simulink model "BlockDiagram_Detailed_Fluids_FirstPrinc"  (R2025b)
settings: Solver=VariableStepAuto  StartTime=0.0  StopTime=10.0  RelTol=1e-3
values from neighbouring files (symbols this model uses):
  c_star_vec = [ ... (first row only)    [cstar_lookup_table.m]
  P_c_vec = 270:350    [a_lookup_table.m]    (also in cstar_lookup_table.m)
undefined symbols (not defined in the file or in its folder): CdA_inj_ox, CdA_max_valve_ox, P_amb, P_feed_f, P_feed_ox, rho_f, rho_ox, V_c
settings Model: Creator=gruby  LastModifiedBy=gruby

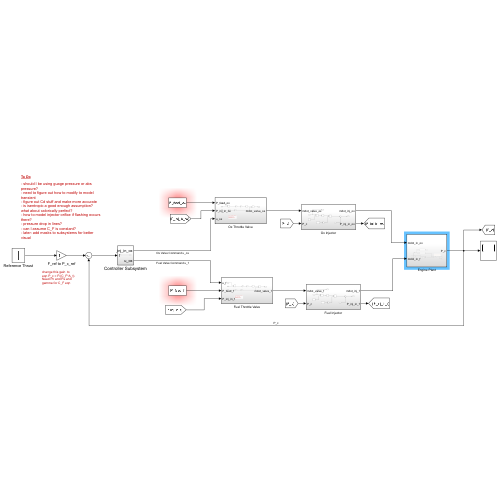
[thumbnail: Simulink's stored preview of the top-level diagram]
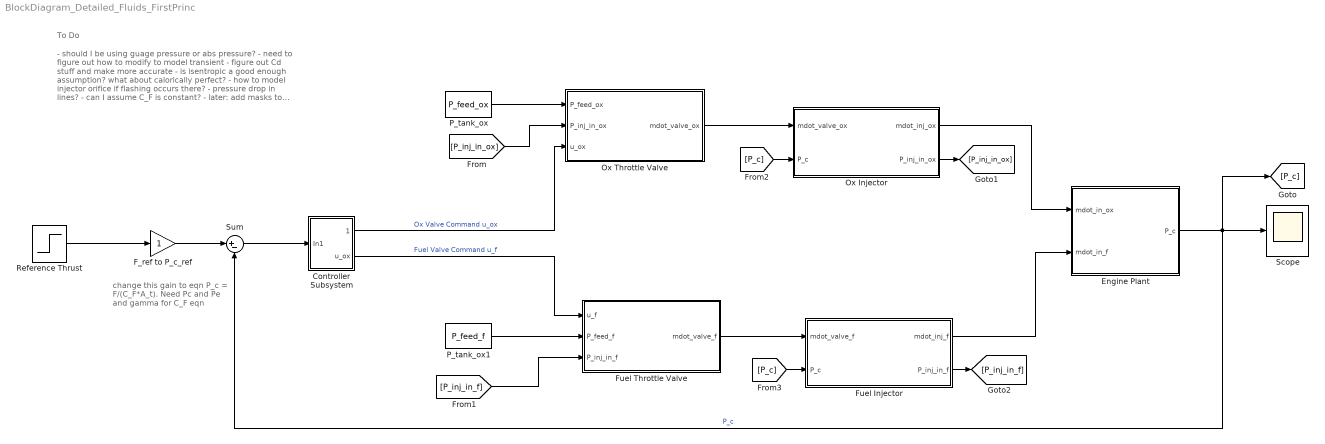
== system BlockDiagram_Detailed_Fluids_FirstPrinc ==
  note: To Do
  note: - should I be using guage pressure or abs pressure?
      | - need to figure out how to modify to model transient
      | - figure out Cd stuff and make more accurate
      | - is isentropic a good enough assumption? what about calorically perfect?
      | - how to model injector orifice if flashing occurs there?
      | - pressure drop in lines?
      | - can I assume C_F is constant?
      | - later: add masks to subsystems for better visual
  note: change this gain to eqn P_c = F/(C_F*A_t). Need Pc and Pe and gamma for C_F eqn
  Controller Subsystem : Subsystem
  Engine Plant : Subsystem
  F_ref to P_c_ref : Gain
  Fuel Injector : Subsystem
  Fuel Throttle Valve : Subsystem
  Ox Injector : Subsystem
  Ox Throttle Valve : Subsystem
  P_tank_ox : Constant  Value=P_feed_ox
  P_tank_ox1 : Constant  Value=P_feed_f
  Reference Thrust : Step  SampleTime=0
  Scope : Scope
      settings: ActiveDisplayYMinimum=-1.8374784378622904  ActiveDisplayYMaximum=16.537497604206919
  Sum : Sum  Inputs=|+-
  wires:
  Sum/1 -> Controller Subsystem/1(In1)
  F_ref to P_c_ref/1 -> Sum/1
  Reference Thrust/1 -> F_ref to P_c_ref/1
  Engine Plant/1(P_c) -> Scope/1, [P_c], Sum/2  "P_c"
  [P_c] -> Ox Injector/2(P_c)
  Controller Subsystem/1(P_inj_in_ox) -> Ox Throttle Valve/3(u_ox)  "Ox Valve Command u_ox"
  P_tank_ox/1 -> Ox Throttle Valve/1(P_feed_ox)
  Ox Throttle Valve/1(mdot_valve_ox) -> Ox Injector/1(mdot_valve_ox)
  Ox Injector/1(mdot_inj_ox) -> Engine Plant/1(mdot_in_ox)
  [P_inj_in_ox] -> Ox Throttle Valve/2(P_inj_in_ox)
  Ox Injector/2(P_inj_in_ox) -> [P_inj_in_ox]
  Controller Subsystem/2(u_ox) -> Fuel Throttle Valve/1(u_f)  "Fuel Valve Command u_f"
  Fuel Injector/2(P_inj_in_f) -> [P_inj_in_f]
  [P_inj_in_f] -> Fuel Throttle Valve/3(P_inj_in_f)
  Fuel Injector/1(mdot_inj_f) -> Engine Plant/2(mdot_in_f)
  [P_c] -> Fuel Injector/2(P_c)
  Fuel Throttle Valve/1(mdot_valve_f) -> Fuel Injector/1(mdot_valve_f)
  P_tank_ox1/1 -> Fuel Throttle Valve/2(P_feed_f)

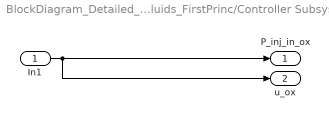
== system BlockDiagram_Detailed_Fluids_FirstPrinc/Controller Subsystem ==
  In1 : Inport
  P_inj_in_ox : Outport
  u_ox : Outport  Port=2
  wires:
  In1/1 -> u_ox/1, P_inj_in_ox/1

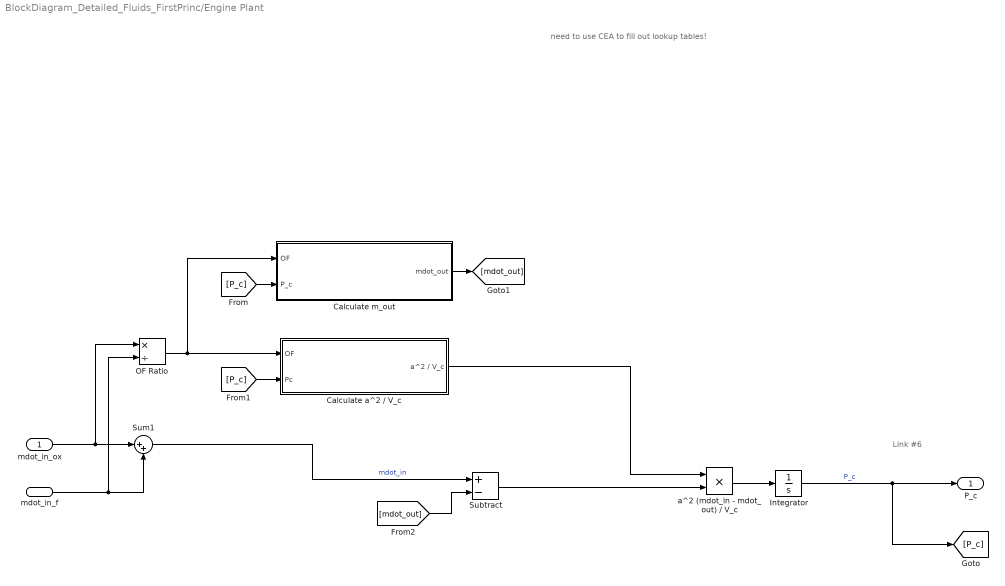
== system BlockDiagram_Detailed_Fluids_FirstPrinc/Engine Plant ==
  note: Link #6
  note: need to use CEA to fill out lookup tables!
  mdot_in_ox : Inport
  mdot_in_f : Inport  Port=2
  Calculate a^2 / V_c : Subsystem
  Calculate m_out : Subsystem
  Integrator : Integrator  InitialCondition=P_amb
  OF Ratio : Product  Inputs=*/
  Subtract : Sum  Inputs=+-
  Sum1 : Sum  Inputs=|++
  "a^2 (mdot_in - mdot_out) / V_c " : Product
  P_c : Outport
  wires:
  mdot_in_f/1 -> OF Ratio/2, Sum1/2
  mdot_in_ox/1 -> OF Ratio/1, Sum1/1
  Integrator/1 -> [P_c], P_c/1  "P_c"
  OF Ratio/1 -> Calculate m_out/1(OF), Calculate a^2 / V_c/1(OF)
  "a^2 (mdot_in - mdot_out) / V_c "/1 -> Integrator/1
  [P_c] -> Calculate m_out/2(P_c)
  [P_c] -> Calculate a^2 / V_c/2(Pc)
  Calculate a^2 / V_c/1(a^2 / V_c) -> "a^2 (mdot_in - mdot_out) / V_c "/1
  Calculate m_out/1(mdot_out) -> [mdot_out]
  Sum1/1 -> Subtract/1  "mdot_in"
  [mdot_out] -> Subtract/2
  Subtract/1 -> "a^2 (mdot_in - mdot_out) / V_c "/2

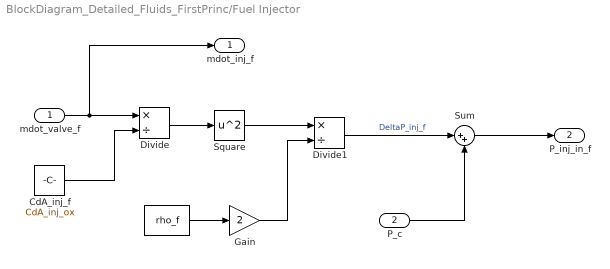
== system BlockDiagram_Detailed_Fluids_FirstPrinc/Fuel Injector ==
  mdot_valve_f : Inport
  P_c : Inport  Port=2
  "   " : Constant  Value=rho_f
  CdA_inj_f : Constant  Value=CdA_inj_ox
  Divide : Product  Inputs=*/
  Divide1 : Product  Inputs=*/
  Gain : Gain  Gain=2
  Square : Math  Operator=square
  Sum : Sum  Inputs=|++
  mdot_inj_f : Outport
  P_inj_in_f : Outport  Port=2
  wires:
  mdot_valve_f/1 -> mdot_inj_f/1, Divide/1
  CdA_inj_f/1 -> Divide/2
  Divide/1 -> Square/1
  Gain/1 -> Divide1/2
  "   "/1 -> Gain/1
  Square/1 -> Divide1/1
  Divide1/1 -> Sum/1  "DeltaP_inj_f"
  P_c/1 -> Sum/2
  Sum/1 -> P_inj_in_f/1

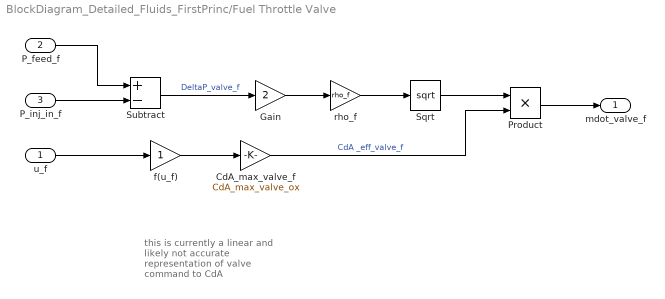
== system BlockDiagram_Detailed_Fluids_FirstPrinc/Fuel Throttle Valve ==
  note: this is currently a linear and likely not accurate representation of valve command to CdA
  u_f : Inport
  P_feed_f : Inport  Port=2
  P_inj_in_f : Inport  Port=3
  CdA_max_valve_f : Gain  Gain=CdA_max_valve_ox
  Gain : Gain  Gain=2
  Product : Product
  Sqrt : Sqrt
  Subtract : Sum  Inputs=+-
  f(u_f) : Gain
  rho_f : Gain  Gain=rho_f
  mdot_valve_f : Outport
  wires:
  f(u_f)/1 -> CdA_max_valve_f/1
  u_f/1 -> f(u_f)/1
  CdA_max_valve_f/1 -> Product/2  "CdA _eff_valve_f"
  P_feed_f/1 -> Subtract/1
  Subtract/1 -> Gain/1  "DeltaP_valve_f"
  Gain/1 -> rho_f/1
  rho_f/1 -> Sqrt/1
  Sqrt/1 -> Product/1
  Product/1 -> mdot_valve_f/1
  P_inj_in_f/1 -> Subtract/2

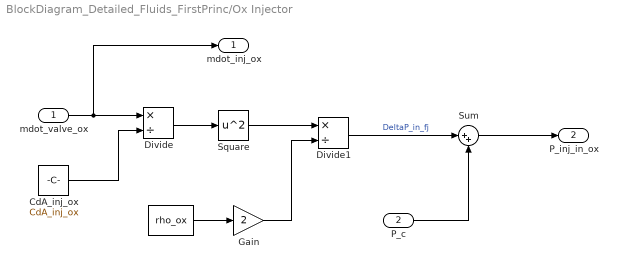
== system BlockDiagram_Detailed_Fluids_FirstPrinc/Ox Injector ==
  mdot_valve_ox : Inport
  P_c : Inport  Port=2
  "   " : Constant  Value=rho_ox
  CdA_inj_ox : Constant  Value=CdA_inj_ox
  Divide : Product  Inputs=*/
  Divide1 : Product  Inputs=*/
  Gain : Gain  Gain=2
  Square : Math  Operator=square
  Sum : Sum  Inputs=|++
  mdot_inj_ox : Outport
  P_inj_in_ox : Outport  Port=2
  wires:
  mdot_valve_ox/1 -> mdot_inj_ox/1, Divide/1
  CdA_inj_ox/1 -> Divide/2
  Divide/1 -> Square/1
  Gain/1 -> Divide1/2
  "   "/1 -> Gain/1
  Square/1 -> Divide1/1
  Divide1/1 -> Sum/1  "DeltaP_in_fj"
  P_c/1 -> Sum/2
  Sum/1 -> P_inj_in_ox/1

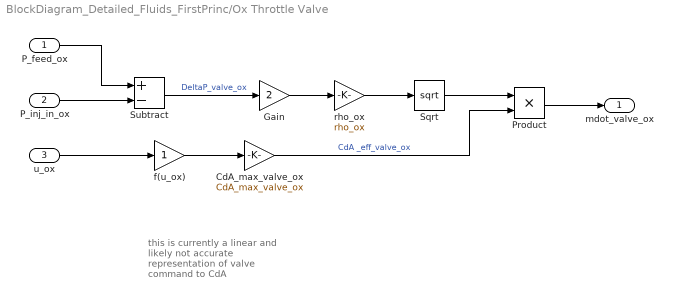
== system BlockDiagram_Detailed_Fluids_FirstPrinc/Ox Throttle Valve ==
  note: this is currently a linear and likely not accurate representation of valve command to CdA
  P_feed_ox : Inport
  P_inj_in_ox : Inport  Port=2
  u_ox : Inport  Port=3
  CdA_max_valve_ox : Gain  Gain=CdA_max_valve_ox
  Gain : Gain  Gain=2
  Product : Product
  Sqrt : Sqrt
  Subtract : Sum  Inputs=+-
  f(u_ox) : Gain
  rho_ox : Gain  Gain=rho_ox
  mdot_valve_ox : Outport
  wires:
  f(u_ox)/1 -> CdA_max_valve_ox/1
  u_ox/1 -> f(u_ox)/1
  CdA_max_valve_ox/1 -> Product/2  "CdA _eff_valve_ox"
  P_feed_ox/1 -> Subtract/1
  Subtract/1 -> Gain/1  "DeltaP_valve_ox"
  Gain/1 -> rho_ox/1
  rho_ox/1 -> Sqrt/1
  Sqrt/1 -> Product/1
  Product/1 -> mdot_valve_ox/1
  P_inj_in_ox/1 -> Subtract/2

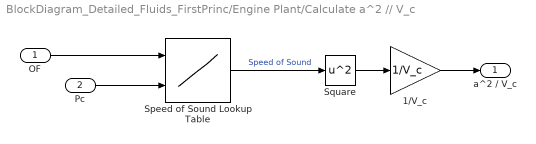
== system BlockDiagram_Detailed_Fluids_FirstPrinc/Engine Plant/Calculate a^2 // V_c ==
  OF : Inport
  Pc : Inport  Port=2
  1/V_c : Gain  Gain=1/V_c
  Speed of Sound Lookup Table : Lookup_n-D  BreakpointsForDimension1=[1:3]  BreakpointsForDimension2=[1:3]  InternalRulePriority=Speed  RndMeth=Simplest
      settings: InputPortMap=u0,u1
  Square : Math  Operator=square
  a^2 / V_c : Outport
  wires:
  Speed of Sound Lookup Table/1 -> Square/1  "Speed of Sound"
  OF/1 -> Speed of Sound Lookup Table/1
  Square/1 -> 1/V_c/1
  Pc/1 -> Speed of Sound Lookup Table/2
  1/V_c/1 -> a^2 / V_c/1

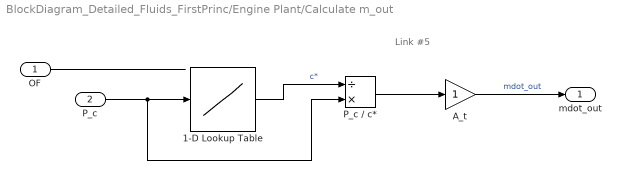
== system BlockDiagram_Detailed_Fluids_FirstPrinc/Engine Plant/Calculate m_out ==
  note: Link #5
  OF : Inport
  P_c : Inport  Port=2
  1-D Lookup Table : Lookup_n-D  NumberOfTableDimensions=1  BreakpointsForDimension1=P_c_vec  Table=c_star_vec  InternalRulePriority=Speed  RndMeth=Simplest
  A_t : Gain
  P_c / c* : Product  Inputs=/*
  mdot_out : Outport
  wires:
  1-D Lookup Table/1 -> P_c / c*/1  "c*"
  P_c / c*/1 -> A_t/1
  OF/1 -> ?
  A_t/1 -> mdot_out/1  "mdot_out"
  P_c/1 -> 1-D Lookup Table/1, P_c / c*/2
